simulink model "T_type_inverter"  (R2024b)
settings: Solver=ode1  StartTime=0.0  StopTime=0.5  FixedStep=1e-6  RelTol=1e-3
libraries: spsIGBTDiodeLib x12, spsDCVoltageSourceLib x2, simulink x2, spsGroundLib x1, spsMultimeterLib x1, spsThreePhaseSeriesRLCLoadLib x1, spsThreePhaseVIMeasurementLib x1, sps_lib x1
settings Model: Creator=killa  LastModifiedBy=killa

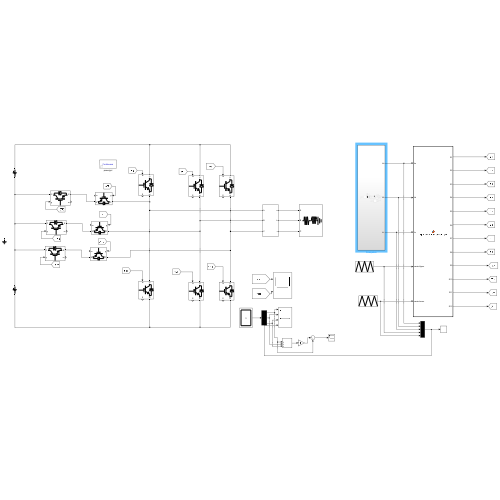
[thumbnail: Simulink's stored preview of the top-level diagram]
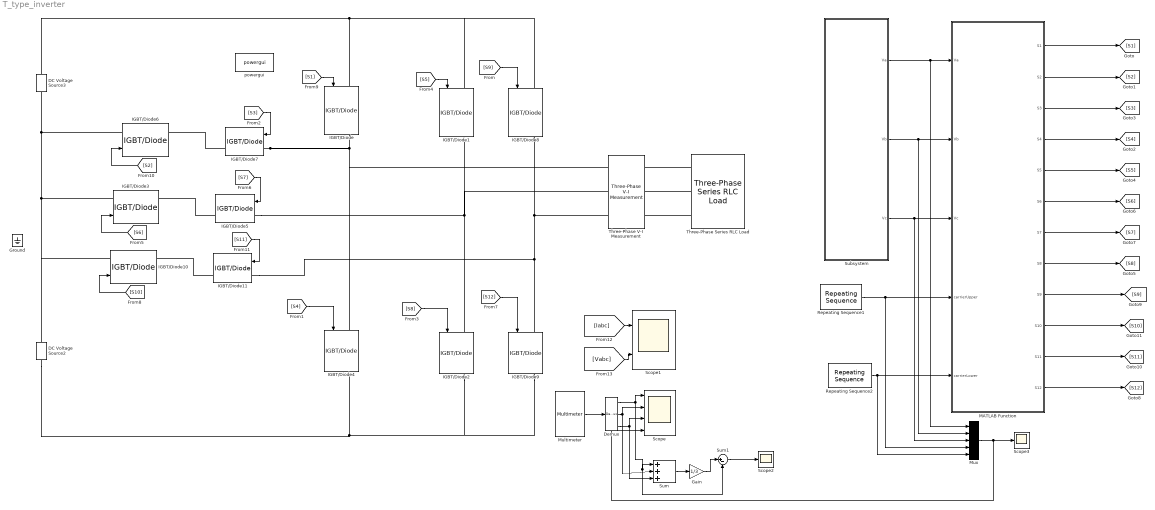
== system T_type_inverter ==
  DC Voltage Source2 : spsDCVoltageSourceLib/DC Voltage Source  Amplitude=300  Measurements=None
  DC Voltage Source3 : spsDCVoltageSourceLib/DC Voltage Source  Amplitude=300  Measurements=None
  Demux : Demux  Outputs=3
  Gain : Gain  Gain=1/3
  Ground : spsGroundLib/Ground  LConnTagsString=a
  IGBT/Diode{,1..11} (12 alike) : spsIGBTDiodeLib/IGBT//Diode  Ron=1e-3  Rs=1e5  Cs=inf  Measurements=on
  MATLAB Function : MATLAB Function  TreatAsAtomicUnit=on
  Multimeter : spsMultimeterLib/Multimeter  L=3  sel=[1 2 3]  yselected={}  Gain=[1 1 1]  OutputType=Complex  PlotAtSimulationStop=off  PhasorSimulation=off
  Mux : Mux  Inputs=5
  Repeating Sequence1 : simulink/Sources/Repeating Sequence  rep_seq_t=[0 0.5 1]/2500  rep_seq_y=[0 1 0]
  Repeating Sequence2 : simulink/Sources/Repeating Sequence  rep_seq_t=[0 0.5 1]/2500  rep_seq_y=[-1 0 -1]
  Scope : Scope  NumInputPorts=4
  Scope1 : Scope  NumInputPorts=2
  Scope2 : Scope
  Scope3 : Scope
  Subsystem : Subsystem
  Sum : Sum  Inputs=|+++
  Sum1 : Sum  Inputs=|+-
  Three-Phase Series RLC Load : spsThreePhaseSeriesRLCLoadLib/Three-Phase Series RLC Load  LConnTagsString=A|B|C  Configuration=Y (grounded)  NominalVoltage=380  Vabc=[1e3 1e3 1e3]  Vabcp=[1e3 1e3 1e3]  NominalFrequency=50  UnbalancedPower=off  ActivePower=5e3  InductivePower=5e3  CapacitivePower=0  Pabc=[10e3 9e3 11e3]  QLabc=[100 90 110]  QCabc=[100 90 110]  Pabcp=[10e3 9e3 11e3]  QLabcp=[100 90 110]  QCabcp=[100 90 110]  Measurements=Branch voltages  LoadType=constant Z
  Three-Phase V-I Measurement : spsThreePhaseVIMeasurementLib/Three-Phase V-I Measurement  VoltageMeasurement=phase-to-phase  SetLabelV=on  LabelV=Vabc  Vpu=off  VpuLL=off  CurrentMeasurement=yes  SetLabelI=on  LabelI=Iabc  Ipu=off  Pbase=100e6  Vbase=500e3  OutputType=Complex  PhasorSimulation=off  PSBequivalent=0
  powergui : sps_lib/powergui  Priority=1  SimulationMode=Continuous  SampleTime=50e-6  frequency=60  Iterations=50  frequencyindice=0  Pbase=100e6  ErrMax=1e-4  UnitsV=kV  UnitsW=MW  buscounter=0  FunctionMessages=off  echomessages=off  EnableUseOfTLC=off  CurrentSourceSwitches=off  DisableSnubberDevices=off  DisableRonSwitches=off  DisableVfSwitches=off  DisplayEquations=off  AutomaticDiscreteSolvers=off  SolverType=Tustin/Backward Euler (TBE)  Interpol=off  ExternalGateDelay=off  methode=off  Ts=100  x0status=blocks  SPID=on  SwTol=0  HookPort=off  NonlinearTolerance=1e-4  nMaxIteration=100  ContinueOnMaxIteration=off  RestoreLinks=warning  ResistiveCurrentMeasurement=off  Frange=[0:2:500]  Ylog=off  Xlog=on  ShowGrid=off  save=off  variable=ZData  structure=0  ZoomFFT=off  StartTime=0.0  cycles=1  DisplayStyle=1  fundamental=60  FreqAxis=off  MaxFrequency=1000  frequencyindicesteady=1  RmsSteady=1  display=off
  wires:
  [S2] -> IGBT/Diode6/1
  [S1] -> IGBT/Diode/1
  [S3] -> IGBT/Diode7/1
  [S4] -> IGBT/Diode4/1
  MATLAB Function/1(S1) -> [S1]
  MATLAB Function/3(S3) -> [S3]
  MATLAB Function/4(S4) -> [S4]
  MATLAB Function/2(S2) -> [S2]
  [S8] -> IGBT/Diode2/1
  [S5] -> IGBT/Diode1/1
  [S6] -> IGBT/Diode3/1
  [S7] -> IGBT/Diode5/1
  [S9] -> IGBT/Diode8/1
  [S12] -> IGBT/Diode9/1
  [S10] -> IGBT/Diode10/1
  [S11] -> IGBT/Diode11/1
  Subsystem/1(Va) -> Mux/1, MATLAB Function/1(Va)
  Subsystem/2(Vb) -> Mux/2, MATLAB Function/2(Vb)
  Subsystem/3(Vc) -> Mux/3, MATLAB Function/3(Vc)
  Repeating Sequence1/1 -> Mux/4, MATLAB Function/4(carrierUpper)
  Repeating Sequence2/1 -> Mux/5, MATLAB Function/5(carrierLower)
  MATLAB Function/5(S5) -> [S5]
  MATLAB Function/8(S8) -> [S8]
  MATLAB Function/6(S6) -> [S6]
  MATLAB Function/7(S7) -> [S7]
  MATLAB Function/9(S9) -> [S9]
  MATLAB Function/10(S10) -> [S10]
  MATLAB Function/11(S11) -> [S11]
  MATLAB Function/12(S12) -> [S12]
  [Iabc] -> Scope1/1
  [Vabc] -> Scope1/2
  Multimeter/1 -> Demux/1
  Demux/1 -> Scope/1, Sum/1, Sum1/2
  Demux/2 -> Sum/2, Scope/2
  Demux/3 -> Sum/3, Scope/3
  Sum/1 -> Gain/1
  Gain/1 -> Sum1/1
  Sum1/1 -> Scope2/1
  Mux/1 -> Scope/4, Scope3/1
  connections:
  DC Voltage Source2/LConn1 -- IGBT/Diode9/RConn1 -- IGBT/Diode2/RConn1 -- IGBT/Diode4/RConn1
  DC Voltage Source3/RConn1 -- IGBT/Diode8/LConn1 -- IGBT/Diode1/LConn1 -- IGBT/Diode/LConn1
  IGBT/Diode7/LConn1 -- IGBT/Diode4/LConn1 -- Three-Phase V-I Measurement/LConn1 -- IGBT/Diode/RConn1
  IGBT/Diode7/RConn1 -- IGBT/Diode6/RConn1
  IGBT/Diode6/LConn1 -- IGBT/Diode10/LConn1 -- DC Voltage Source2/RConn1 -- IGBT/Diode3/LConn1 -- DC Voltage Source3/LConn1
  IGBT/Diode2/LConn1 -- Three-Phase V-I Measurement/LConn2 -- IGBT/Diode1/RConn1 -- IGBT/Diode5/LConn1
  IGBT/Diode5/RConn1 -- IGBT/Diode3/RConn1
  IGBT/Diode9/LConn1 -- Three-Phase V-I Measurement/LConn3 -- IGBT/Diode8/RConn1 -- IGBT/Diode11/LConn1
  IGBT/Diode11/RConn1 -- IGBT/Diode10/RConn1
  Three-Phase Series RLC Load/LConn1 -- Three-Phase V-I Measurement/RConn1
  Three-Phase Series RLC Load/LConn2 -- Three-Phase V-I Measurement/RConn2
  Three-Phase Series RLC Load/LConn3 -- Three-Phase V-I Measurement/RConn3

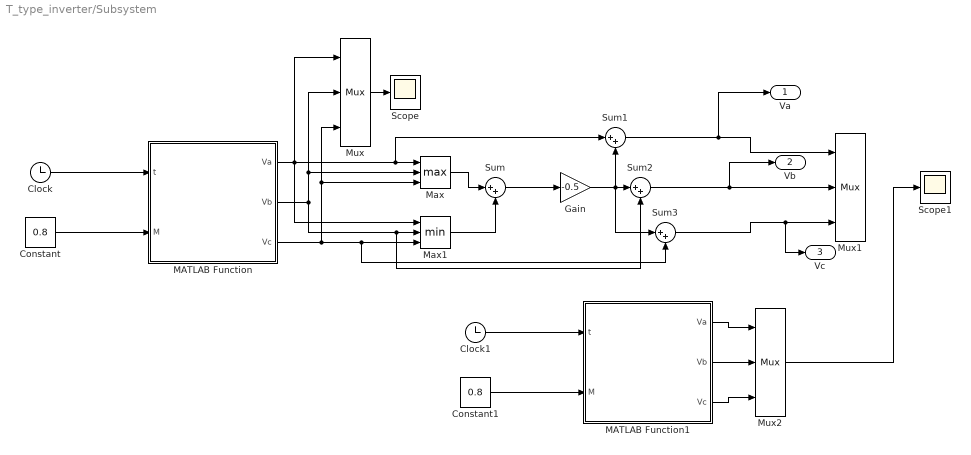
== system T_type_inverter/Subsystem ==
  Clock : Clock
  Clock1 : Clock
  Constant : Constant  Value=0.8
  Constant1 : Constant  Value=0.8
  Gain : Gain  Gain=-0.5
  MATLAB Function : MATLAB Function  TreatAsAtomicUnit=on
  MATLAB Function1 : MATLAB Function  TreatAsAtomicUnit=on
  Max : MinMax  Function=max  Inputs=3
  Max1 : MinMax  Inputs=3
  Mux : Mux  Inputs=3
  Mux1 : Mux  Inputs=3
  Mux2 : Mux  Inputs=3
  Scope : Scope
  Scope1 : Scope
  Sum{,1..3} (4 alike) : Sum  Inputs=|++
  Va : Outport
  Vb : Outport  Port=2
  Vc : Outport  Port=3
  wires:
  Sum1/1 -> Va/1, Mux1/1
  MATLAB Function/1(Va) -> Max1/1, Sum1/1, Max/1, Mux/1
  MATLAB Function/2(Vb) -> Max/2, Mux/2, Sum2/2, Max1/2
  Sum3/1 -> Vc/1, Mux1/3
  MATLAB Function/3(Vc) -> Sum3/2, Max1/3, Max/3, Mux/3
  Constant/1 -> MATLAB Function/2(M)
  Mux/1 -> Scope/1
  Gain/1 -> Sum3/1, Sum2/1, Sum1/2
  Max1/1 -> Sum/2
  Sum/1 -> Gain/1
  Max/1 -> Sum/1
  Clock/1 -> MATLAB Function/1(t)
  Sum2/1 -> Vb/1, Mux1/2
  Constant1/1 -> MATLAB Function1/2(M)
  Clock1/1 -> MATLAB Function1/1(t)
  MATLAB Function1/1(Va) -> Mux2/1
  MATLAB Function1/2(Vb) -> Mux2/2
  MATLAB Function1/3(Vc) -> Mux2/3
  Mux2/1 -> Scope1/1

== matlab function T_type_inverter/Subsystem/MATLAB Function1 ==
  data: t input; Va output; M input; Vb output; Vc output
function [Va, Vb, Vc] = fcn(t,M)

% Shift only the negative half-cycle upward by +1
f = 50;          % Fundamental frequency (Hz)         % Modulation index (Amplitude)

% Angular frequency
w = 2*pi*f;

% Three-phase sine waves
Va = M*sin(w*t);
Vb = M*sin(w*t - 2*pi/3);   % -120 degrees
Vc = M*sin(w*t + 2*pi/3);   % +120 degrees



end

== matlab function T_type_inverter/Subsystem/MATLAB Function ==
  data: t input; Va output; M input; Vb output; Vc output
function [Va, Vb, Vc] = fcn(t,M)

% Shift only the negative half-cycle upward by +1
f = 50;          % Fundamental frequency (Hz)         % Modulation index (Amplitude)

% Angular frequency
w = 2*pi*f;

% Three-phase sine waves
Va = M*sin(w*t);
Vb = M*sin(w*t - 2*pi/3);   % -120 degrees
Vc = M*sin(w*t + 2*pi/3);   % +120 degrees



end

== matlab function T_type_inverter/MATLAB Function ==
  data: Va input; Vb input; Vc input; S1 output; S2 output; S3 output; S4 output; carrierUpper input; carrierLower input; S5 output; S6 output; S7 output; S8 output; S9 output; S10 output; S11 output; S12 output
function [S1,S2,S3,S4,S5,S6,S7,S8,S9,S10,S11,S12] = ...
    ttype_pwm_dual_carrier_3ph(Va, Vb, Vc, carrierUpper, carrierLower)
% Va, Vb, Vc    : raw reference sines, range -1 to 1, 120 deg apart
% carrierUpper  : triangular carrier, range 0 to 1  (shared by all 3 phases)
% carrierLower  : triangular carrier, range -1 to 0  (shared by all 3 phases)

%========================
% Phase A
%========================
S1 = Va >= carrierUpper;   % ">=" block
S3 = ~S1;                   % NOT gate, top branch
S4 = Va <= carrierLower;   % "<=" block
S2 = ~S4;                   % NOT gate, bottom branch

%========================
% Phase B
%========================
S5 = Vb >= carrierUpper;
S7 = ~S5;
S8 = Vb <= carrierLower;
S6 = ~S8;

%========================
% Phase C
%========================
S9  = Vc >= carrierUpper;
S11 = ~S9;
S12 = Vc <= carrierLower;
S10 = ~S12;
